simulink model "DC_motor_realtime_test_quad_reward_noisdone_criteria"  (R2021a)
settings: Solver=VariableStepAuto  StartTime=0.0  StopTime=inf  RelTol=1e-3
undefined symbols (not defined in the file or in its folder): DiscIntNeverNeededParam
libraries: rllib x1
settings Model: Creator=SHRENI MALYALA  LastModifiedBy=SHRENI MALYALA

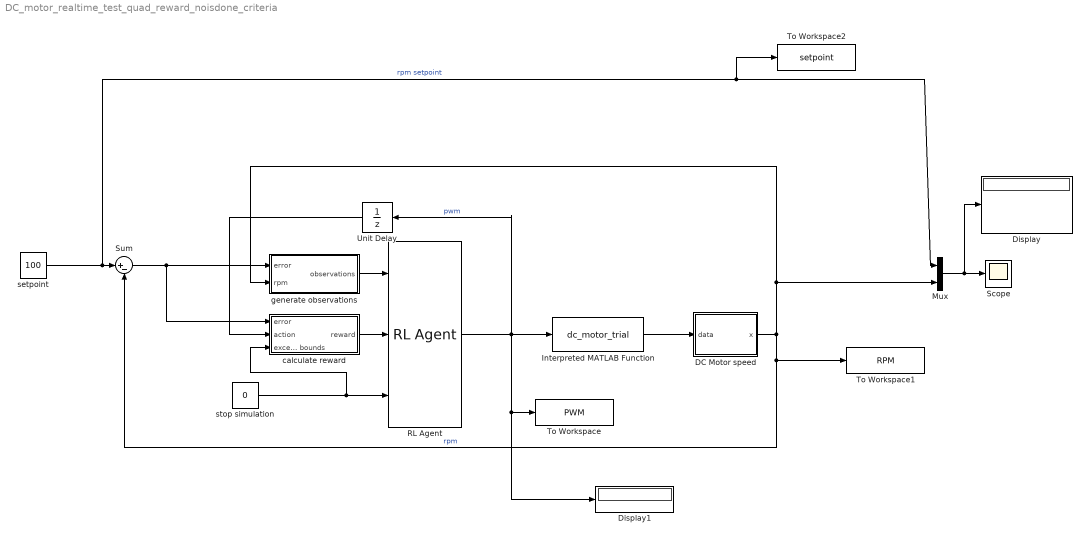
== system DC_motor_realtime_test_quad_reward_noisdone_criteria ==
  "DC Motor speed " : MATLAB Function  TreatAsAtomicUnit=on
  Display : Display
  Display1 : Display
  Interpreted MATLAB Function : MATLABFcn  MATLABFcn=dc_motor_trial  OutputDimensions=[1,2]  Output1D=off
  Mux : Mux  Inputs=2
  RL Agent : rllib/RL Agent  Agent=agent  ExternalActionAsInput=off  ProvideCumRwd=off  TreatAsDirectFeedthrough=on
  Scope : Scope
  Sum : Sum  Inputs=|+-
  To Workspace : ToWorkspace  VariableName=PWM  SaveFormat=Timeseries  SampleTime=-1
  To Workspace1 : ToWorkspace  VariableName=RPM  SaveFormat=Timeseries  SampleTime=-1
  To Workspace2 : ToWorkspace  VariableName=setpoint  SaveFormat=Timeseries  SampleTime=-1
  Unit Delay : UnitDelay  SampleTime=-1  HasFrameUpgradeWarning=on
  calculate reward : Subsystem
  generate observations : Subsystem
  setpoint : Constant  Value=100  SampleTime=0.015
  stop simulation : Constant  Value=0
  wires:
  generate observations/1(observations) -> RL Agent/1
  calculate reward/1(reward) -> RL Agent/2
  stop simulation/1 -> calculate reward/3(exceed bounds), RL Agent/3
  setpoint/1 -> To Workspace2/1, Mux/1, Sum/1  "rpm setpoint"
  Sum/1 -> calculate reward/1(error), generate observations/1(error)
  RL Agent/1 -> To Workspace/1, Display1/1, Unit Delay/1, Interpreted MATLAB Function/1  "pwm"
  Interpreted MATLAB Function/1 -> "DC Motor speed "/1(data)
  "DC Motor speed "/1(x) -> Mux/2, generate observations/2(rpm), Sum/2, To Workspace1/1  "rpm"
  Mux/1 -> Display/1, Scope/1
  Unit Delay/1 -> calculate reward/2(action)

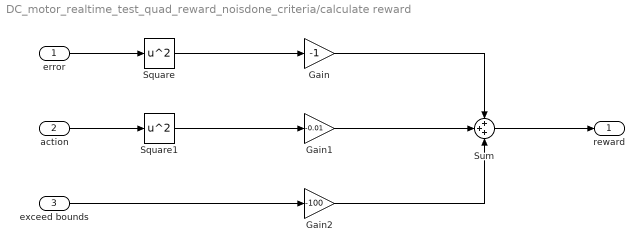
== system DC_motor_realtime_test_quad_reward_noisdone_criteria/calculate reward ==
  error : Inport
  action : Inport  Port=2
  exceed bounds : Inport  Port=3
  Gain : Gain  Gain=-1
  Gain1 : Gain  Gain=-0.01
  Gain2 : Gain  Gain=-100
  Square : Math  Operator=square  SaturateOnIntegerOverflow=on
  Square1 : Math  Operator=square  SaturateOnIntegerOverflow=on
  Sum : Sum  Inputs=+++
  reward : Outport
  wires:
  error/1 -> Square/1
  Square/1 -> Gain/1
  action/1 -> Square1/1
  Square1/1 -> Gain1/1
  exceed bounds/1 -> Gain2/1
  Gain/1 -> Sum/1
  Gain1/1 -> Sum/2
  Gain2/1 -> Sum/3
  Sum/1 -> reward/1

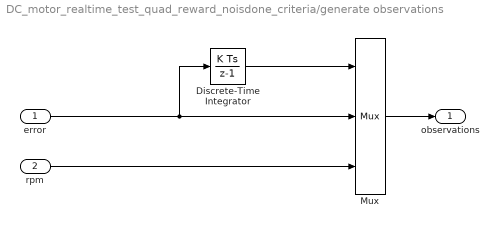
== system DC_motor_realtime_test_quad_reward_noisdone_criteria/generate observations ==
  error : Inport
  rpm : Inport  Port=2
  Discrete-Time Integrator : DiscreteIntegrator  SampleTime=-1  ICPrevOutput=DiscIntNeverNeededParam  ICPrevScaledInput=DiscIntNeverNeededParam
  Mux : Mux  Inputs=3
  observations : Outport
  wires:
  error/1 -> Discrete-Time Integrator/1, Mux/2
  rpm/1 -> Mux/3
  Discrete-Time Integrator/1 -> Mux/1
  Mux/1 -> observations/1

== matlab function DC_motor_realtime_test_quad_reward_noisdone_criteria/DC Motor speed  ==
  data: data input; x output
function x  = PWM(data)

F = data(:,1)*256;
r = data(:,2);
x = (F+r)*8.982025;

end
